simulink model "Mechanical_SMD_System"  (R2023b)
settings: Solver=VariableStepAuto  StartTime=0.0  StopTime=150  MaxStep=0.01  RelTol=1e-3
model workspace (MAT data in the model file):
  b = 0.5
  k = 1
  m = 10
settings Model: Creator=91839  LastModifiedBy=siva kumar
settings SolverCC: AlgebraicLoopSolver=TrustRegion
settings DataIOCC: ExternalInput=data  SaveFormat=Array  DSMLogging=off  ReturnWorkspaceOutputs=off
settings DebuggingCC: UnconnectedInputMsg=warning  UnconnectedOutputMsg=warning  UnconnectedLineMsg=warning
settings ModelReferenceCC: EnableRefExpFcnMdlSchedulingChecks=on
settings SFSimCC: CustomCodeUndefinedFunction=UseInterfaceOnly

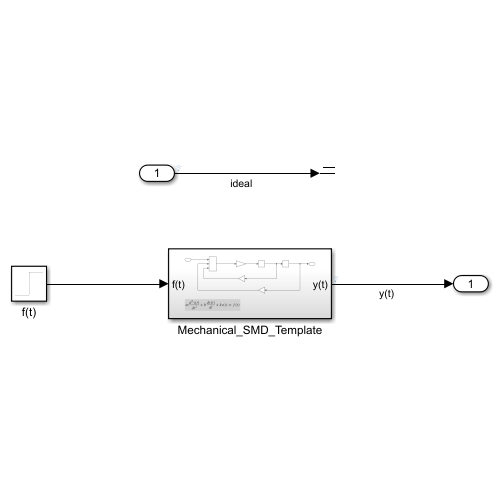
[thumbnail: Simulink's stored preview of the top-level diagram]
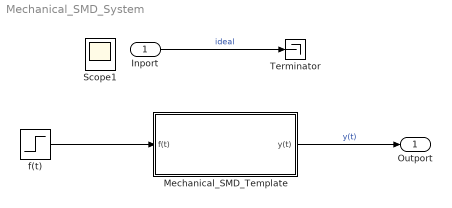
== system Mechanical_SMD_System ==
  Inport : Inport
  Mechanical_SMD_Template : Subsystem
  Terminator : Terminator
  f(t) : Step  SampleTime=0
  Outport : Outport
  Scope1 : Scope
  wires:
  Inport/1 -> Terminator/1  "ideal"
  f(t)/1 -> Mechanical_SMD_Template/1(f(t))
  Mechanical_SMD_Template/1(y(t)) -> Outport/1  "y(t)"

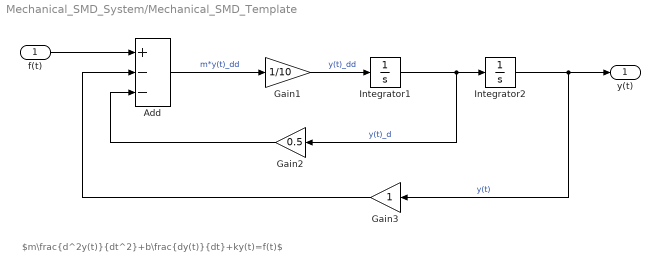
== system Mechanical_SMD_System/Mechanical_SMD_Template ==
  note: $m\frac{d^2y(t)}{dt^2}+b\frac{dy(t)}{dt}+ky(t)=f(t)$
  f(t) : Inport
  Add : Sum  Inputs=+--
  Gain1 : Gain  Gain=1/10
  Gain2 : Gain  Gain=0.5
  Gain3 : Gain
  Integrator1 : Integrator
  Integrator2 : Integrator  InitialCondition=1.8
  y(t) : Outport
  wires:
  Add/1 -> Gain1/1  "m*y(t)_dd"
  Gain1/1 -> Integrator1/1  "y(t)_dd"
  Integrator1/1 -> Integrator2/1, Gain2/1  "y(t)_d"
  Integrator2/1 -> y(t)/1, Gain3/1  "y(t)"
  Gain2/1 -> Add/3
  Gain3/1 -> Add/2
  f(t)/1 -> Add/1
